simulink library "Softclipper"  (R2022b)
settings: Solver=VariableStepAuto  StartTime=0.0  StopTime=10.0  RelTol=1e-3
libraries: SoftclipperBtc x1
settings Model: Creator=jb10849  LastModifiedBy=kl13806
settings SolverCC: AlgebraicLoopSolver=TrustRegion
settings DebuggingCC: UnconnectedInputMsg=warning  UnconnectedOutputMsg=warning  UnconnectedLineMsg=warning  SFMachineParentedDataDiag=warning  ArithmeticOperatorsInVariantConditions=warning
settings ModelReferenceCC: EnableRefExpFcnMdlSchedulingChecks=on
settings SFSimCC: SimUseLocalCustomCode=off  CustomCodeUndefinedFunction=UseInterfaceOnly
settings RTWCC: RTWUseLocalCustomCode=off  DLArmComputeVersion=19.05

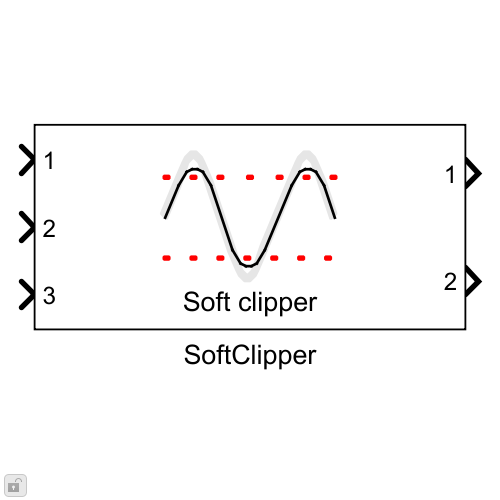
[thumbnail: Simulink's stored preview of the top-level diagram]
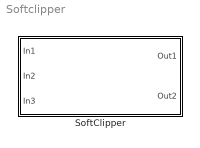
== system Softclipper ==
  SoftClipper : Subsystem  mask{MaskXmin=[], MaskYMax=[], MaxXminLow=[], MaskYMaxLow=[]}
      mask prompts: MaskXmin "xmin"; MaskYMax "ymax"; MaxXminLow "xmin low"; MaskYMaxLow "ymax low"
      mask init:
      | blkh = gcbh;
      | % Copy discrete mask parameters into a classdef object
      | InnerLinkConfig = SoftClipperConfig;
      | InnerLinkConfig.DefaultXmin = MaskXmin;
      | InnerLinkConfig.DefaultYmax = MaskYMax;
      | InnerLinkConfig.DefaultXminLow = MaxXminLow;
      | InnerLinkConfig.DefaultYmaxLow = MaskYMaxLow;
      mask DialogControl Container3 Prompt: Parameter Set 1
      mask DialogControl Container6 Prompt: Parameter Set 2 (for start-stop situation)
      mask Display:
      | [path,w,h] = IconSoftclipperMask();
      | 
      | % work in pixels since the icon does not scale
      | pos = get(gcbh,'position');
      | bw = pos(3) - pos(1);
      | bh = pos(4) - pos(2);
      | 
      | % Draw centered icon
      | xAdj = bw/2 - w/2;
      | yAdj = bh/2 - h/2 + 4;
      | for i=1:length(path)
      |     if (path(i).rgb(1) >= 0)
      |         patch(path(i).x+xAdj, path(i).y+yAdj, path(i).rgb);
      |     end
      |     if (path(i).stroke(1) >= 0)
      |         plot(path(i).x+xAdj, path(i).y+yAdj);
      |     end
      | end
      | 
      | % Anchor the corners of the coordinate system
      | patch(0,0,[1 1 1]);
      | patch(bw,bh,[1 1 1]);
      | 
      | % Display some text
      | text(bw/2, 4,'Soft clipper', ...
      |     'horizontalAlignment','center', ...
      |     'VerticalAlignment','bottom');

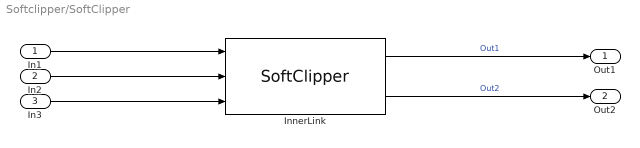
== system Softclipper/SoftClipper ==
  In1 : Inport
  In2 : Inport  Port=2
  In3 : Inport  Port=3
  InnerLink : SoftclipperBtc/SoftClipper  Config=InnerLinkConfig  FeatureName=Sclip
      settings: SourceProductName=Bose Blocklib
  Out1 : Outport
  Out2 : Outport  Port=2
  wires:
  InnerLink/1 -> Out1/1  "Out1"
  InnerLink/2 -> Out2/1  "Out2"
  In1/1 -> InnerLink/1
  In2/1 -> InnerLink/2
  In3/1 -> InnerLink/3
